simulink model "Waypoints_Controller_Observer"  (R2025b)
settings: Solver=VariableStepAuto  StartTime=0.0  StopTime=120  RelTol=1e-3
values from neighbouring files (symbols this model uses):
  Aobs = [p.A_lin-L*C]    [drone_controller_with_observer.m]
  Bobs = [p.B_lin L]    [drone_controller_with_observer.m]
undefined symbols (not defined in the file or in its folder): K, p
libraries: simulink x2, discretizing x1
settings Model: Creator=chako  LastModifiedBy=chako

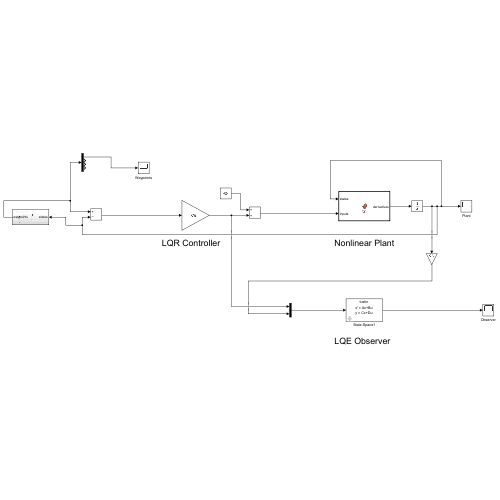
[thumbnail: Simulink's stored preview of the top-level diagram]
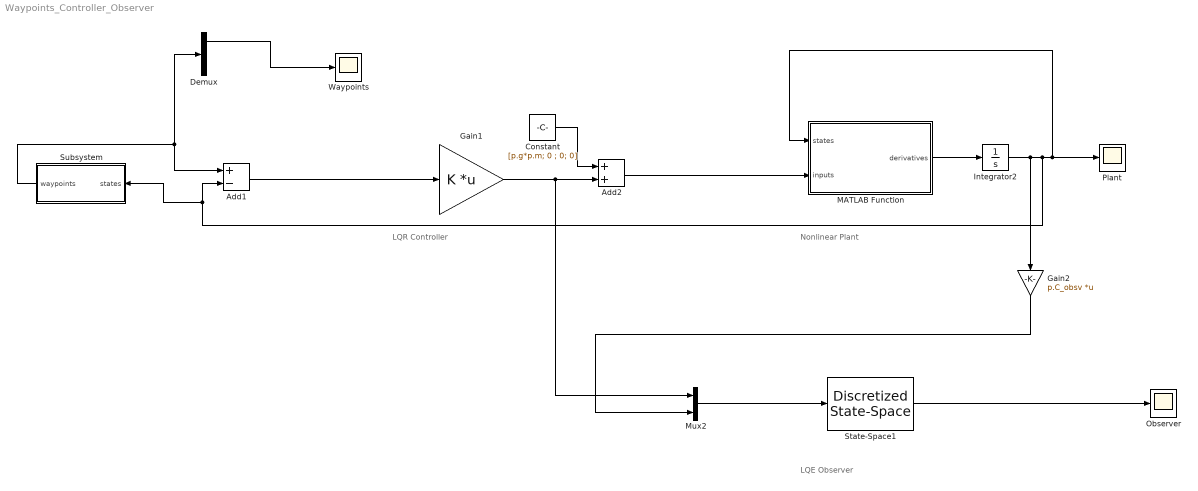
== system Waypoints_Controller_Observer ==
  note: Nonlinear Plant
  note: LQR Controller
  note: LQE Observer
  Add1 : Sum  Inputs=+-
  Add2 : Sum
  Constant : Constant  Value=[p.g*p.m; 0 ; 0; 0]
  Demux : Demux
  Gain1 : Gain  Gain=K  Multiplication=Matrix(K*u)
  Gain2 : Gain  Gain=p.C_obsv  Multiplication=Matrix(K*u)
  Integrator2 : Integrator  InitialCondition=[0;0;0;0;0;0;0;0;0;0;0;0]
  MATLAB Function : MATLAB Function  TreatAsAtomicUnit=on
  Mux2 : Mux  Inputs=2
  Observer : Scope
      settings: ActiveDisplayYMinimum=-9.5284442079811846  ActiveDisplayYMaximum=9.0802014412009235  DataLoggingVariableName=ScopeData3
  Plant : Scope
      settings: ActiveDisplayYMinimum=-13.272021598503848  ActiveDisplayYMaximum=13.768800180707615  DataLoggingVariableName=ScopeData2
  State-Space1 : discretizing/Discretized State-Space  A=Aobs  B=Bobs  C=eye(12)  D=zeros(12, 10)  ic=0  AbsTol=auto  SampleTime=0.01  method=tustin  Wc=1
  Subsystem : Subsystem
  Waypoints : Scope
      settings: DataLoggingVariableName=ScopeData5
  wires:
  Gain1/1 -> Mux2/1, Add2/2
  Add2/1 -> MATLAB Function/2(inputs)
  Constant/1 -> Add2/1
  MATLAB Function/1(derivatives) -> Integrator2/1
  Add1/1 -> Gain1/1
  State-Space1/1 -> Observer/1
  Mux2/1 -> State-Space1/1
  Gain2/1 -> Mux2/2
  Integrator2/1 -> Gain2/1, Add1/2, Subsystem/1(states), MATLAB Function/1(states), Plant/1
  Subsystem/1(waypoints) -> Demux/1, Add1/1
  Demux/1 -> Waypoints/1

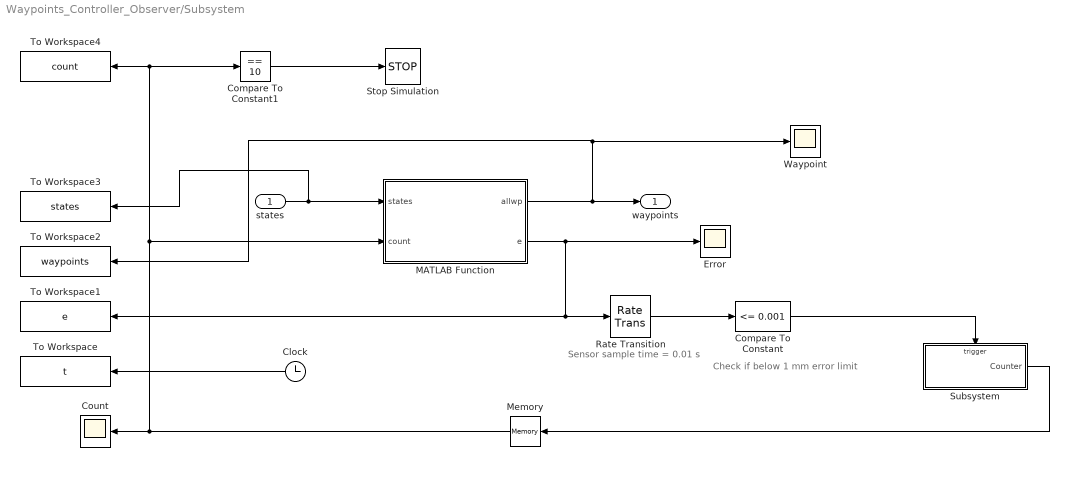
== system Waypoints_Controller_Observer/Subsystem ==
  note: Sensor sample time = 0.01 s
  note: Check if below 1 mm error limit
  states : Inport
  Clock : Clock
  Compare To Constant : simulink/Logic and Bit Operations/Compare To Constant  relop=<=  const=0.001  OutDataTypeStr=boolean
  Compare To Constant1 : simulink/Logic and Bit Operations/Compare To Constant  relop===  const=10  OutDataTypeStr=boolean
  Count : Scope
      settings: ActiveDisplayYMinimum=-16.093302218045451  ActiveDisplayYMaximum=19.823824302397149  DataLoggingVariableName=ScopeData4
  Error : Scope
  MATLAB Function : MATLAB Function  TreatAsAtomicUnit=on
  Memory : Memory  InheritSampleTime=on
  Rate Transition : RateTransition  OutPortSampleTime=0.01
  Stop Simulation : Stop
  Subsystem : Subsystem
  To Workspace : ToWorkspace  VariableName=t  SampleTime=-1
  To Workspace1 : ToWorkspace  VariableName=e  SampleTime=-1
  To Workspace2 : ToWorkspace  VariableName=waypoints  SampleTime=-1
  To Workspace3 : ToWorkspace  VariableName=states  SampleTime=-1
  To Workspace4 : ToWorkspace  VariableName=count  SampleTime=-1
  Waypoint : Scope
  waypoints : Outport
  wires:
  states/1 -> To Workspace3/1, MATLAB Function/1(states)
  MATLAB Function/2(e) -> Rate Transition/1, To Workspace1/1, Error/1
  Rate Transition/1 -> Compare To Constant/1
  Memory/1 -> MATLAB Function/2(count), Compare To Constant1/1, To Workspace4/1, Count/1
  Clock/1 -> To Workspace/1
  MATLAB Function/1(allwp) -> waypoints/1, To Workspace2/1, Waypoint/1
  Compare To Constant1/1 -> Stop Simulation/1
  Subsystem/1(Counter) -> Memory/1
  Compare To Constant/1 -> Subsystem/Trigger

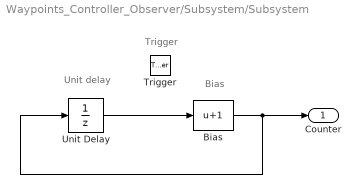
== system Waypoints_Controller_Observer/Subsystem/Subsystem ==
  note: Unit delay
  note: Bias
  note: Trigger
  Trigger : TriggerPort  VariantControl=(inherit)  InitialTriggerSignalState=positive  PortDimensions=1
  Bias : Bias  Bias=1  SaturateOnIntegerOverflow=off
  Unit Delay : UnitDelay  SampleTime=-1  HasFrameUpgradeWarning=on
  Counter : Outport  PortDimensions=[1,1]
  wires:
  Bias/1 -> Unit Delay/1, Counter/1
  Unit Delay/1 -> Bias/1

== matlab function Waypoints_Controller_Observer/Subsystem/MATLAB Function ==
  data: states input size=12; allwp output size=12; count input size=1; p parameter; e output
function [allwp, e] = waypoints(states, count, p)

allwp = zeros(12, 1); % 12 parameters of interest
wp = zeros(3, 1); % 3 physical waypoints (x, y, z)
xi = states(1:3); % initial position values (x, y, z)

if count < 10
    wp = p.wp(:, (count+1));
    disp(count)
    disp(",")
    disp(wp)
    disp("-------------")
else
    % wp(1) = 9 * cos(0.2*pi*t);
    % wp(2) = 9 * sin(0.2*pi*t);
    % wp(3) = 5 + 0.1 *sin(0.4*pi*t);
    wp(1) = 0;
    wp(2) = 0;
    wp(3) = 0;
end
e = norm(xi-wp);

allwp (1:3) = wp;
allwp (4:12) = 0;

== matlab function Waypoints_Controller_Observer/MATLAB Function ==
  data: states input size=12; derivatives output size=12; inputs input size=4; p parameter
function derivatives = fcn(states, inputs, p)

 % I is the inertia matrix
    I = [p.Ixx 0 0;
         0 p.Iyy 0;
         0 0 p.Izz];

    xi= states(1:3); % x, y, z
    xid = states(4:6); %x_prime, y_prime, z_prime
    eta = states(7:9); % roll, pitch, yaw
    etad = states(10:12); % roll_prime, pitch_prime, yaw_prime

    % Cosines of each
    c_roll = cos(eta(1));
    c_pitch = cos(eta(2));
    c_yaw = cos(eta(3));

    % Sines of each
    s_roll = sin(eta(1));
    s_pitch = sin(eta(2));
    s_yaw = sin(eta(3));


    % Derivative of xi is xid

    % Calculative derivatives of xid
    xidd = [0;0;-p.g] - (p.kD/p.m)*xid + ...
        ([s_roll*s_yaw + c_roll*s_pitch*c_yaw;
         c_roll*s_pitch*s_yaw - s_roll*c_yaw;
         c_roll*c_pitch]*inputs(1))*1/p.m; % Dividing by m here


    % Derivative of eta is etad
    % Calculative derivatives of etad


    % eta is [phi, theta, psi] = roll pitch yaw
    W = [1  0       -s_pitch;
         0  c_roll  s_roll * c_pitch;
         0 -s_roll  c_roll * c_pitch];
    % v is rpy in body frame
    
    tau_body = [inputs(2);
                inputs(3);
                inputs(4)];
    v = W * etad;
    vd = inv(I) * (tau_body + [(p.Iyy - p.Izz)*v(2)*v(3); ... 
                               (p.Izz - p.Ixx)*v(1)*v(3);
                               (p.Ixx - p.Iyy)*v(1)*v(2)]);
    Wd = [0        0                  -etad(2)*cos(-etad(2));
          0 -etad(1)*s_roll            etad(1)*c_roll*c_pitch;
          0 -etad(1)*c_roll -etad(1)*s_roll*c_pitch-etad(2)*c_roll*s_pitch];
    etadd = inv(W) * (vd - Wd*etad);
    derivatives = [xid; xidd; etad; etadd];
end
